simulink model "behinesazislx"  (R2018b)
settings: Solver=VariableStepAuto  StartTime=0.0  StopTime=10  FixedStep=0.01  RelTol=1e-5
values from neighbouring files (symbols this model uses):
  A = double(A)    [Linearization.m]    (also in findK_emtiazi.m = [1 2 0; 0 -1 3; 0 1 -1])
  B = double(B)    [Linearization.m]
  C = [1 0 0 0 ; 0 1 0 0 ]    [Linearization.m]    (also in findK_emtiazi.m = [0 1 0])
  k1 = double(k1)    [Linearization.m]
settings Model: Creator=Mr.Hallajiyan  LastModifiedBy=sepehr
settings DebuggingCC: LibraryContextMissingDiagnostic=none
settings SFSimCC: SimUseLocalCustomCode=off
settings RTWCC: RTWUseLocalCustomCode=off

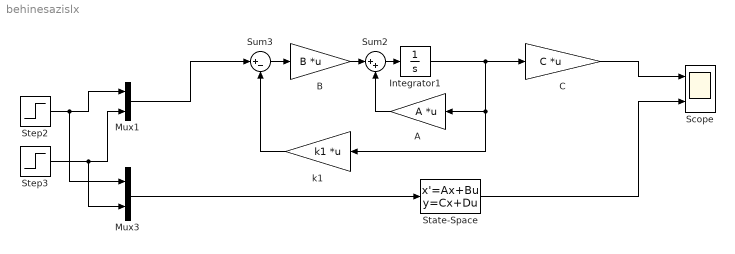
== system behinesazislx ==
  "A " : Gain  Gain=A  Multiplication=Matrix(K*u) (u vector)
  B : Gain  Gain=B  Multiplication=Matrix(K*u) (u vector)
  C : Gain  Gain=C  Multiplication=Matrix(K*u) (u vector)
  Integrator1 : Integrator  InitialCondition=[0.5;0.5;0.005;0.008]  IgnoreLimit=on
  Mux1 : Mux  Inputs=2
  Mux3 : Mux  Inputs=2
  Scope : Scope  NumInputPorts=2
  State-Space : StateSpace  A=A  B=B  C=C  D=zeros(2)  InitialCondition=[0.5;0.5;0;0]
  Step2 : Step  After=100  SampleTime=0.1
  Step3 : Step  After=100  SampleTime=0.1
  Sum2 : Sum  Inputs=|++
  Sum3 : Sum  Inputs=|+-
  "k1 " : Gain  Gain=k1  Multiplication=Matrix(K*u) (u vector)
  wires:
  Step3/1 -> Mux1/2, Mux3/2
  Step2/1 -> Mux3/1, Mux1/1
  Sum2/1 -> Integrator1/1
  B/1 -> Sum2/1
  "A "/1 -> Sum2/2
  "k1 "/1 -> Sum3/2
  Sum3/1 -> B/1
  Mux3/1 -> State-Space/1
  Mux1/1 -> Sum3/1
  State-Space/1 -> Scope/2
  C/1 -> Scope/1
  Integrator1/1 -> C/1, "A "/1, "k1 "/1
